simulink model "conSys_2robots_5_vR2014a"  (Simulink 8.3)
settings: Solver=FixedStepDiscrete  StartTime=0.0  StopTime=200  FixedStep=Ts  RelTol=1e-3
values from neighbouring files (symbols this model uses):
  ck = double(max(abs([par.q0_r1;par.q0_r2] - [par.q0r_r1;par.q0r_r2]))*20/7000 + 6)    [startUp_conSys_2robots_1_vGPU_vR2014a.m]    (also in startUp_conSys_2robots_1_vR2014a.m = max(abs([par.q0_r1;par.q0_r2] - [par.q0r_r1;par.q0r_r2]))*20; startUp_conSys_2robots_2_vR2014a.m = max(abs([par.q0_r1;par.q0_r2] - [par.q0r_r1;par.q0r_r2]))*20; startUp_conSys_2robots_3_vR2014a.m = max(abs([par.q0_r1;par.q0_r2] - [par.q0r_r1;par.q0r_r2]))*20; startUp_conSys_2robots_4_vR2014a.m = max(abs([par.q0_r1;par.q0_r2] - [par.q0r_r1;par.q0r_r2]))*20)
  d_0 = 2000    [startUp_conSys_2robots_1_vGPU_vR2014a.m]    (also in startUp_conSys_2robots_1_vR2014a.m = 200; startUp_conSys_2robots_2_vR2014a.m = 200; startUp_conSys_2robots_3_vR2014a.m; startUp_conSys_2robots_4_vR2014a.m = 200)
  do1r_0 = dthc_0 + dph1_0    (= 0.2)    [startUp_conSys_2robots_1_vGPU_vR2014a.m]    (also in startUp_conSys_2robots_1_vR2014a.m = 0; startUp_conSys_2robots_2_vR2014a.m = 0; startUp_conSys_2robots_3_vR2014a.m = 0; startUp_conSys_2robots_4_vR2014a.m = 0)
  do2r_0 = dthc_0 + dph2_0    (= -0.2)    [startUp_conSys_2robots_1_vGPU_vR2014a.m]    (also in startUp_conSys_2robots_1_vR2014a.m = 0; startUp_conSys_2robots_2_vR2014a.m = 0; startUp_conSys_2robots_3_vR2014a.m = 0; startUp_conSys_2robots_4_vR2014a.m = 0)
  dx1r_0 = dxc_0 + sin(thc_0)*dd_0 + d_0*cos(thc_0)*dthc_0    [startUp_conSys_2robots_1_vGPU_vR2014a.m]    (also in startUp_conSys_2robots_1_vR2014a.m; startUp_conSys_2robots_2_vR2014a.m; startUp_conSys_2robots_3_vR2014a.m; startUp_conSys_2robots_4_vR2014a.m)
  dx2r_0 = dxc_0 - sin(thc_0)*dd_0 - d_0*cos(thc_0)*dthc_0    [startUp_conSys_2robots_1_vGPU_vR2014a.m]    (also in startUp_conSys_2robots_1_vR2014a.m; startUp_conSys_2robots_2_vR2014a.m; startUp_conSys_2robots_3_vR2014a.m; startUp_conSys_2robots_4_vR2014a.m)
  dy1r_0 = dyc_0 + cos(thc_0)*dd_0 - d_0*sin(thc_0)*dthc_0    [startUp_conSys_2robots_1_vGPU_vR2014a.m]    (also in startUp_conSys_2robots_1_vR2014a.m; startUp_conSys_2robots_2_vR2014a.m; startUp_conSys_2robots_3_vR2014a.m; startUp_conSys_2robots_4_vR2014a.m)
  dy2r_0 = dyc_0 - cos(thc_0)*dd_0 + d_0*sin(thc_0)*dthc_0    [startUp_conSys_2robots_1_vGPU_vR2014a.m]    (also in startUp_conSys_2robots_1_vR2014a.m; startUp_conSys_2robots_2_vR2014a.m; startUp_conSys_2robots_3_vR2014a.m; startUp_conSys_2robots_4_vR2014a.m)
  o1r_0 = pi/2 - thc_0    (= 0)    [startUp_conSys_2robots_1_vGPU_vR2014a.m]    (also in startUp_conSys_2robots_1_vR2014a.m = pi/2 - thc_0; startUp_conSys_2robots_2_vR2014a.m = pi/2 - thc_0; startUp_conSys_2robots_3_vR2014a.m; startUp_conSys_2robots_4_vR2014a.m = th1_0)
  o2r_0 = pi/2 - thc_0    (= 0)    [startUp_conSys_2robots_1_vGPU_vR2014a.m]    (also in startUp_conSys_2robots_1_vR2014a.m = pi/2 - thc_0; startUp_conSys_2robots_2_vR2014a.m = pi/2 - thc_0; startUp_conSys_2robots_3_vR2014a.m; startUp_conSys_2robots_4_vR2014a.m = th2_0)
  thc_0 = pi/2    (= 1.57079632679)    [startUp_conSys_2robots_1_vGPU_vR2014a.m]    (also in startUp_conSys_2robots_1_vR2014a.m = atan2(1/25,1/12.5) + pi/2; startUp_conSys_2robots_2_vR2014a.m = atan2(1/25,1/12.5) + pi/2; startUp_conSys_2robots_3_vR2014a.m; startUp_conSys_2robots_4_vR2014a.m = atan2(1/25,1/12.5) + pi/2)
  Ts = 1/200    (= 0.005)    [startUp_conSys_2robots_1_vGPU_vR2014a.m]    (also in startUp_conSys_2robots_1_vR2014a.m = 0.0125; startUp_conSys_2robots_2_vR2014a.m = 0.01; startUp_conSys_2robots_3_vR2014a.m; startUp_conSys_2robots_4_vR2014a.m)
  x1_0 = 12000    [startUp_conSys_2robots_1_vGPU_vR2014a.m]    (also in startUp_conSys_2robots_1_vR2014a.m = 13178.9; startUp_conSys_2robots_2_vR2014a.m = 13178.9; startUp_conSys_2robots_3_vR2014a.m; startUp_conSys_2robots_4_vR2014a.m = 13178.9)
  x2_0 = 8000    [startUp_conSys_2robots_1_vGPU_vR2014a.m]    (also in startUp_conSys_2robots_1_vR2014a.m = 12821.1; startUp_conSys_2robots_2_vR2014a.m = 12821.1; startUp_conSys_2robots_3_vR2014a.m; startUp_conSys_2robots_4_vR2014a.m = 12821.1)
  xc_0 = 10000    [startUp_conSys_2robots_1_vGPU_vR2014a.m]    (also in startUp_conSys_2robots_1_vR2014a.m = 13000; startUp_conSys_2robots_2_vR2014a.m = 13000; startUp_conSys_2robots_3_vR2014a.m; startUp_conSys_2robots_4_vR2014a.m = 13000)
  y1_0 = 10000    [startUp_conSys_2robots_1_vGPU_vR2014a.m]    (also in startUp_conSys_2robots_1_vR2014a.m = 12910.6; startUp_conSys_2robots_2_vR2014a.m = 12910.6; startUp_conSys_2robots_3_vR2014a.m; startUp_conSys_2robots_4_vR2014a.m = 12910.6)
  y2_0 = 10000    [startUp_conSys_2robots_1_vGPU_vR2014a.m]    (also in startUp_conSys_2robots_1_vR2014a.m = 13089.4; startUp_conSys_2robots_2_vR2014a.m = 13089.4; startUp_conSys_2robots_3_vR2014a.m; startUp_conSys_2robots_4_vR2014a.m = 13089.4)
  yc_0 = 10000    [startUp_conSys_2robots_1_vGPU_vR2014a.m]    (also in startUp_conSys_2robots_1_vR2014a.m = 13000; startUp_conSys_2robots_2_vR2014a.m = 13000; startUp_conSys_2robots_3_vR2014a.m; startUp_conSys_2robots_4_vR2014a.m = 13000)
undefined symbols (not defined in the file or in its folder): absoluteAngle01_vR2014a, absoluteAngle02_vR2014a, absoluteAngle03_vR2014a, absoluteAngle04_vR2014a, absoluteAngle05_vR2014a, absoluteAngle06_vR2014a, absoluteAngle07_vR2014a, DiscIntNeverNeededParam
undefined symbols (not defined in the file): ADAMS_cwd, ADAMS_exec, ADAMS_host, ADAMS_init, ADAMS_inputs, ADAMS_outputs, ADAMS_prefix, ADAMS_static, ADAMS_sysdir
libraries: simulink x18, cstblocks x1
(part 1 of 2)
settings Model: Creator=baqumau  LastModifiedBy=mauro
settings DataIOCC: SignalLoggingSaveFormat=Dataset
settings DebuggingCC: UnderspecifiedInitializationDetection=Simplified  StateNameClashWarn=none
settings GRTTargetCC: CombineOutputUpdateFcns=on  GRTInterface=off

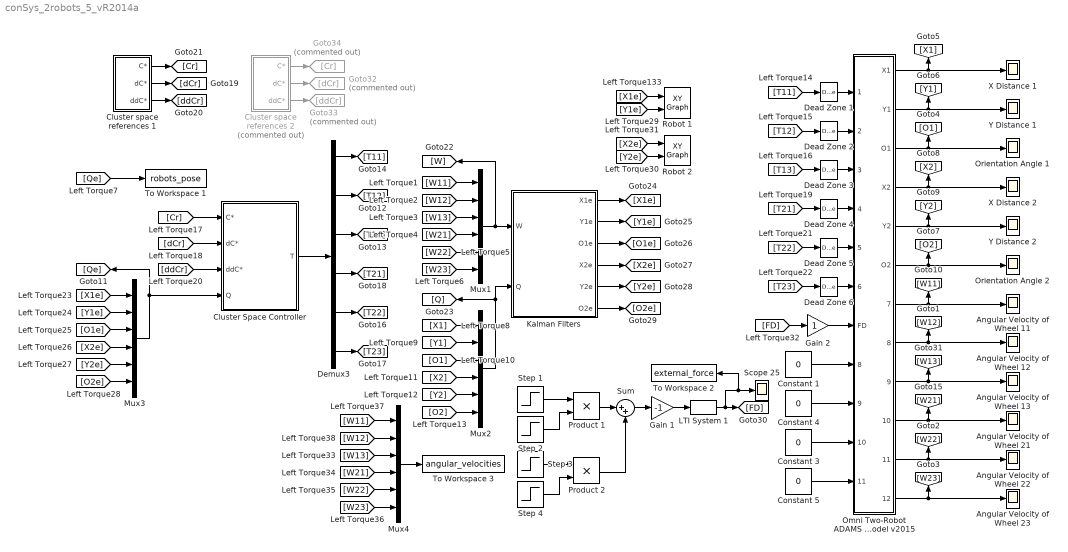
== system conSys_2robots_5_vR2014a ==
  Angular Velocity of Wheel {11..13,21..23} (6 alike) : Scope
      Angular Velocity of Wheel 11 settings: YMin=-20  YMax=20  SaveName=ScopeData3
      Angular Velocity of Wheel 12 settings: YMin=-200  YMax=20  SaveName=ScopeData6
      Angular Velocity of Wheel 13 settings: YMin=-10  YMax=20  SaveName=ScopeData9
      Angular Velocity of Wheel 21 settings: YMin=-20  YMax=20  SaveName=ScopeData2
      Angular Velocity of Wheel 22 settings: YMin=-15  YMax=18  SaveName=ScopeData10
      Angular Velocity of Wheel 23 settings: YMin=-15  YMax=15  SaveName=ScopeData11
  Cluster Space Controller : Subsystem
  Cluster space references 1 : Subsystem
  Cluster space references 2 : Subsystem  Commented=on
  Constant {1,3..5} (4 alike) : Constant  Value=0
  Dead Zone {1..6} (6 alike) : DeadZone  LowerValue=-25  UpperValue=25  SaturateOnIntegerOverflow=on
  Demux3 : Demux  Outputs=6
  Gain 1 : Gain  Gain=-1
  Gain 2 : Gain
  Goto32 : Goto  Commented=on  GotoTag=dCr
  Goto33 : Goto  Commented=on  GotoTag=ddCr
  Goto34 : Goto  Commented=on  GotoTag=Cr
  Kalman Filters : Subsystem
  LTI System 1 : cstblocks/LTI System  sys=Fz  IC=[]
  Mux{1..4} (4 alike) : Mux  Inputs=6
  Omni Two-Robot ADAMS Model v2015 : Subsystem
  Orientation Angle 1 : Scope
  Orientation Angle 2 : Scope
      settings: YMin=-3  YMax=3  SaveName=ScopeData12
  Product 1 : Product
  Product 2 : Product
  Robot 1 : simulink/Sinks/XY Graph  xmin=0  xmax=20000  ymin=0  ymax=20000  st=-1
  Robot 2 : simulink/Sinks/XY Graph  xmin=0  xmax=20000  ymin=0  ymax=20000  st=-1
  Scope 25 : Scope
      settings: YMin=-6  YMax=6  SaveName=ScopeData36
  Step 1 : Step  Time=60  SampleTime=0
  Step 2 : Step  Time=100  Before=1  After=0  SampleTime=0
  Step 3 : Step  Time=130  After=-1  SampleTime=0
  Step 4 : Step  Time=170  Before=1  After=0  SampleTime=0
  Sum : Sum  Inputs=|++
  To Workspace 1 : ToWorkspace  VariableName=robots_pose  SaveFormat=Structure With Time  SampleTime=-1
  To Workspace 2 : ToWorkspace  VariableName=external_force  SaveFormat=Structure With Time  SampleTime=-1
  To Workspace 3 : ToWorkspace  VariableName=angular_velocities  SaveFormat=Structure With Time  SampleTime=-1
  X Distance 1 : Scope
      settings: YMin=0  YMax=20000  SaveName=ScopeData4
  X Distance 2 : Scope
      settings: YMin=0  YMax=20000  SaveName=ScopeData16
  Y Distance 1 : Scope
      settings: YMin=0  YMax=20000
  Y Distance 2 : Scope
      settings: YMin=0  YMax=20000  SaveName=ScopeData17
  wires:
  Omni Two-Robot ADAMS Model v2015/1(X1) -> X Distance 1/1, [X1]
  Omni Two-Robot ADAMS Model v2015/2(Y1) -> [Y1], Y Distance 1/1
  Omni Two-Robot ADAMS Model v2015/3(O1) -> [O1], Orientation Angle 1/1
  Omni Two-Robot ADAMS Model v2015/7(W11) -> [W11], Angular Velocity of Wheel 11/1
  Omni Two-Robot ADAMS Model v2015/10(W21) -> [W21], Angular Velocity of Wheel 21/1
  Omni Two-Robot ADAMS Model v2015/9(W13) -> Angular Velocity of Wheel 13/1, [W13]
  Omni Two-Robot ADAMS Model v2015/4(X2) -> X Distance 2/1, [X2]
  Omni Two-Robot ADAMS Model v2015/5(Y2) -> Y Distance 2/1, [Y2]
  Omni Two-Robot ADAMS Model v2015/6(O2) -> Orientation Angle 2/1, [O2]
  Omni Two-Robot ADAMS Model v2015/8(W12) -> Angular Velocity of Wheel 12/1, [W12]
  Omni Two-Robot ADAMS Model v2015/11(W22) -> Angular Velocity of Wheel 22/1, [W22]
  Omni Two-Robot ADAMS Model v2015/12(W23) -> [W23], Angular Velocity of Wheel 23/1
  [O1e] -> Mux3/3
  [X2e] -> Mux3/4
  [Y2e] -> Mux3/5
  [O2e] -> Mux3/6
  [X1e] -> Mux3/1
  [Y1e] -> Mux3/2
  [Cr] -> Cluster Space Controller/1(C*)
  [dCr] -> Cluster Space Controller/2(dC*)
  Mux3/1 -> Cluster Space Controller/4(Q), [Qe]
  Cluster Space Controller/1(T) -> Demux3/1
  Demux3/1 -> [T11]
  Demux3/2 -> [T12]
  Demux3/3 -> [T13]
  Demux3/4 -> [T21]
  Demux3/5 -> [T22]
  Demux3/6 -> [T23]
  Cluster space references 1/1(C*) -> [Cr]
  Cluster space references 1/2(dC*) -> [dCr]
  Cluster space references 1/3(ddC*) -> [ddCr]
  [ddCr] -> Cluster Space Controller/3(ddC*)
  [W13] -> Mux1/3
  [W21] -> Mux1/4
  [W22] -> Mux1/5
  [W23] -> Mux1/6
  [W11] -> Mux1/1
  [W12] -> Mux1/2
  Mux1/1 -> Kalman Filters/1(W), [W]
  [Qe] -> To Workspace 1/1
  [O1] -> Mux2/3
  [X2] -> Mux2/4
  [Y2] -> Mux2/5
  [O2] -> Mux2/6
  [X1] -> Mux2/1
  [Y1] -> Mux2/2
  Kalman Filters/1(X1e) -> [X1e]
  Kalman Filters/2(Y1e) -> [Y1e]
  Kalman Filters/3(O1e) -> [O1e]
  Kalman Filters/4(X2e) -> [X2e]
  Kalman Filters/5(Y2e) -> [Y2e]
  Kalman Filters/6(O2e) -> [O2e]
  [T11] -> Dead Zone 1/1
  [T12] -> Dead Zone 2/1
  [T13] -> Dead Zone 3/1
  [T21] -> Dead Zone 4/1
  [T22] -> Dead Zone 5/1
  [T23] -> Dead Zone 6/1
  [FD] -> Gain 2/1
  Constant 1/1 -> Omni Two-Robot ADAMS Model v2015/8(FX1)
  Constant 3/1 -> Omni Two-Robot ADAMS Model v2015/10(FY1)
  Constant 4/1 -> Omni Two-Robot ADAMS Model v2015/9(FX2)
  Constant 5/1 -> Omni Two-Robot ADAMS Model v2015/11(FY2)
  [X1e] -> Robot 1/1
  [Y1e] -> Robot 1/2
  [X2e] -> Robot 2/1
  [Y2e] -> Robot 2/2
  Step 1/1 -> Product 1/1
  Step 2/1 -> Product 1/2
  Step 3/1 -> Product 2/1
  Step 4/1 -> Product 2/2
  Product 1/1 -> Sum/1
  Product 2/1 -> Sum/2
  Sum/1 -> Gain 1/1
  LTI System 1/1 -> To Workspace 2/1, Scope 25/1, [FD]
  Gain 1/1 -> LTI System 1/1
  Cluster space references 2/1(C*) -> Goto34/1
  Cluster space references 2/2(dC*) -> Goto32/1
  Cluster space references 2/3(ddC*) -> Goto33/1
  [W13] -> Mux4/3
  [W21] -> Mux4/4
  [W22] -> Mux4/5
  [W23] -> Mux4/6
  [W11] -> Mux4/1
  [W12] -> Mux4/2
  Mux4/1 -> To Workspace 3/1
  Mux2/1 -> Kalman Filters/2(Q), [Q]
  Gain 2/1 -> Omni Two-Robot ADAMS Model v2015/7(FD)
  Dead Zone 1/1 -> Omni Two-Robot ADAMS Model v2015/1(T11)
  Dead Zone 2/1 -> Omni Two-Robot ADAMS Model v2015/2(T12)
  Dead Zone 3/1 -> Omni Two-Robot ADAMS Model v2015/3(T13)
  Dead Zone 4/1 -> Omni Two-Robot ADAMS Model v2015/4(T21)
  Dead Zone 5/1 -> Omni Two-Robot ADAMS Model v2015/5(T22)
  Dead Zone 6/1 -> Omni Two-Robot ADAMS Model v2015/6(T23)

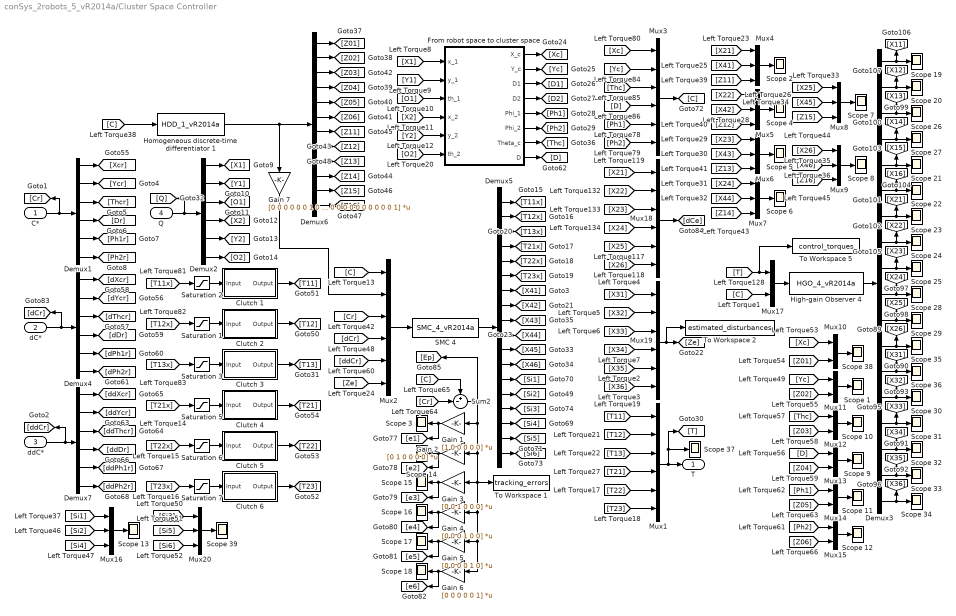
== system conSys_2robots_5_vR2014a/Cluster Space Controller ==
  C* : Inport
  dC* : Inport  Port=2
  ddC* : Inport  Port=3
  Q : Inport  Port=4
  Clutch 1 : Subsystem
  Clutch 2 : Subsystem
  Clutch 3 : Subsystem
  Clutch 4 : Subsystem
  Clutch 5 : Subsystem
  Clutch 6 : Subsystem
  Demux{1..2,4,7} (4 alike) : Demux  Outputs=6
  Demux3 : Demux  Outputs=18
  Demux5 : Demux  Outputs=18
  Demux6 : Demux  Outputs=12
  From robot space to cluster space : Subsystem
  Gain 1 : Gain  Gain=[1 0 0 0 0 0]  Multiplication=Matrix(K*u)
  Gain 2 : Gain  Gain=[0 1 0 0 0 0]  Multiplication=Matrix(K*u)
  Gain 3 : Gain  Gain=[0 0 1 0 0 0]  Multiplication=Matrix(K*u)
  Gain 4 : Gain  Gain=[0 0 0 1 0 0]  Multiplication=Matrix(K*u)
  Gain 5 : Gain  Gain=[0 0 0 0 1 0]  Multiplication=Matrix(K*u)
  Gain 6 : Gain  Gain=[0 0 0 0 0 1]  Multiplication=Matrix(K*u)
  Gain 7 : Gain  Gain=[0 0 0 0 0 0 1 0 0 0 0 0;0 0 0 0 0 0 0 1 0 0 0 0;0 0 0 0 0 0 0 0 1 0 0 0;0 0 0 0 0 0 0 0 0 1 0 0;0 0 0 0 0 0 0 0 0 0 1 0;0 0 0 0 0 0 0 0 0 0 0 1]  Multiplication=Matrix(K*u)
  High-gain Observer 4 : S-Function  FunctionName=HGO_4_vR2014a  Parameters=par  EnableBusSupport=off
  Homogeneous discrete-time differentiator 1 : S-Function  FunctionName=HDD_1_vR2014a  Parameters=par  EnableBusSupport=off
  Mux{1..3,18..19} (5 alike) : Mux  Inputs=6
  Mux{10..15,17} (7 alike) : Mux  Inputs=2
  Mux{4..9,16,20} (8 alike) : Mux  Inputs=3
  SMC 4 : S-Function  FunctionName=SMC_4_vR2014a  Parameters=par  EnableBusSupport=off
  Saturation {1..3,5..7} (6 alike) : Saturate  UpperLimit=100  LowerLimit=-100
  Scope {1..39} (39 alike) : Scope
      Scope 1 settings: YMin=0  YMax=15000  SaveName=ScopeData21
      Scope 10 settings: SaveName=ScopeData39
      Scope 11 settings: SaveName=ScopeData43
      Scope 12 settings: SaveName=ScopeData44
      Scope 13 settings: YMin=-2000  YMax=1000  SaveName=ScopeData45
      Scope 14 settings: YMin=-5000  YMax=1000  SaveName=ScopeData77
      Scope 15 settings: YMin=-4  YMax=4  SaveName=ScopeData78
      Scope 16 settings: YMin=-2000  YMax=2000  SaveName=ScopeData82
      Scope 17 settings: SaveName=ScopeData83
      Scope 18 settings: SaveName=ScopeData84
      Scope 19 settings: YMin=-2000  YMax=16000  SaveName=ScopeData86
      Scope 2 settings: YMin=0  YMax=140  SaveName=ScopeData22
      Scope 20 settings: YMin=0  YMax=20000  SaveName=ScopeData87
      Scope 21 settings: YMin=0  YMax=5000  SaveName=ScopeData88
      Scope 22 settings: YMin=-100  YMax=200  SaveName=ScopeData90
      Scope 23 settings: YMin=-10  YMax=100  SaveName=ScopeData91
      Scope 24 settings: YMin=-50  YMax=50  SaveName=ScopeData92
      Scope 25 settings: YMin=-6  YMax=6  SaveName=ScopeData93
      Scope 26 settings: SaveName=ScopeData94
      Scope 27 settings: TimeRange=388  YMin=-1000  YMax=1000  SaveName=ScopeData95
      Scope 28 settings: YMin=-5000  YMax=1000  SaveName=ScopeData96
      Scope 29 settings: YMin=-10  YMax=10  SaveName=ScopeData97
      Scope 3 settings: YMin=-5000  YMax=3000  SaveName=ScopeData40
      Scope 30 settings: YMin=-1000  YMax=1000  SaveName=ScopeData98
      Scope 31 settings: YMin=-2  YMax=2  SaveName=ScopeData99
      Scope 32 settings: YMin=-1000  YMax=500  SaveName=ScopeData100
      Scope 33 settings: YMin=-6  YMax=8  SaveName=ScopeData101
      Scope 34 settings: YMin=-4  YMax=4  SaveName=ScopeData102
      Scope 35 settings: SaveName=ScopeData103
      Scope 36 settings: YMin=-1000  YMax=500  SaveName=ScopeData104
      Scope 37 settings: YMin=-100  YMax=100  SaveName=ScopeData119
      Scope 38 settings: YMin=0  YMax=15000  SaveName=ScopeData46
      Scope 39 settings: YMin=-15  YMax=15  SaveName=ScopeData47
      Scope 4 settings: YMin=-100  YMax=100  SaveName=ScopeData23
      Scope 5 settings: YMin=-1  YMax=1  SaveName=ScopeData24
      Scope 6 settings: YMin=-1000  YMax=1000  SaveName=ScopeData30
      Scope 7 settings: SaveName=ScopeData31
      Scope 8 settings: YMin=-10  YMax=10  SaveName=ScopeData37
      Scope 9 settings: YMin=500  YMax=10000  SaveName=ScopeData41
  Sum2 : Sum  Inputs=+-|
  To Workspace 1 : ToWorkspace  VariableName=tracking_errors  SaveFormat=Structure With Time  SampleTime=-1
  To Workspace 2 : ToWorkspace  VariableName=estimated_disturbances  SaveFormat=Structure With Time  SampleTime=-1
  To Workspace 5 : ToWorkspace  VariableName=control_torques  SaveFormat=Structure With Time  SampleTime=-1
  T : Outport
  wires:
  Q/1 -> Demux2/1, [Q]
  Demux2/1 -> [X1]
  Demux2/2 -> [Y1]
  Demux2/3 -> [O1]
  Demux2/4 -> [X2]
  Demux2/5 -> [Y2]
  Demux2/6 -> [O2]
  Mux2/1 -> SMC 4/1
  Demux5/1 -> [T11x]
  Demux5/2 -> [T12x]
  Demux5/3 -> [T13x]
  SMC 4/1 -> Demux5/1
  Demux5/4 -> [T21x]
  Demux5/5 -> [T22x]
  Demux5/6 -> [T23x]
  [Cr] -> Sum2/2
  [C] -> Sum2/1
  [T11x] -> Saturation 2/1
  Clutch 1/1(Output) -> [T11]
  [T12x] -> Saturation 1/1
  Clutch 2/1(Output) -> [T12]
  [T13x] -> Saturation 3/1
  Clutch 3/1(Output) -> [T13]
  [T21x] -> Saturation 5/1
  Clutch 4/1(Output) -> [T21]
  [T22x] -> Saturation 6/1
  Clutch 5/1(Output) -> [T22]
  [T23x] -> Saturation 7/1
  Clutch 6/1(Output) -> [T23]
  [T11] -> Mux1/1
  [T23] -> Mux1/6
  [T21] -> Mux1/4
  [T22] -> Mux1/5
  [T12] -> Mux1/2
  [T13] -> Mux1/3
  Mux1/1 -> [T], Scope 37/1, T/1
  C*/1 -> [Cr], Demux1/1
  Demux1/1 -> [Xcr]
  Demux1/2 -> [Ycr]
  Demux1/3 -> [Thcr]
  Demux1/4 -> [Dr]
  Demux1/5 -> [Ph1r]
  Demux1/6 -> [Ph2r]
  dC*/1 -> [dCr], Demux4/1
  Demux4/1 -> [dXcr]
  Demux4/2 -> [dYcr]
  Demux4/3 -> [dThcr]
  Demux4/4 -> [dDr]
  Demux4/5 -> [dPh1r]
  Demux4/6 -> [dPh2r]
  Demux7/1 -> [ddXcr]
  Demux7/2 -> [ddYcr]
  Demux7/3 -> [ddThcr]
  Demux7/4 -> [ddDr]
  Demux7/5 -> [ddPh1r]
  Demux7/6 -> [ddPh2r]
  ddC*/1 -> [ddCr], Demux7/1
  [Xc] -> Mux3/1
  [Ph2] -> Mux3/6
  [D] -> Mux3/4
  [Ph1] -> Mux3/5
  [Yc] -> Mux3/2
  [Thc] -> Mux3/3
  Mux3/1 -> [C]
  Gain 1/1 -> [e1], Scope 3/1
  Gain 2/1 -> [e2], Scope 14/1
  Gain 3/1 -> [e3], Scope 15/1
  Gain 4/1 -> [e4], Scope 16/1
  Gain 5/1 -> [e5], Scope 17/1
  Sum2/1 -> [Ep], To Workspace 1/1, Gain 6/1, Gain 5/1, Gain 4/1, Gain 3/1, Gain 2/1, Gain 1/1
  Gain 6/1 -> [e6], Scope 18/1
  Mux17/1 -> High-gain Observer 4/1
  Demux3/9 -> Scope 25/1, [X23]
  Demux3/7 -> [X21], Scope 23/1
  Demux3/8 -> [X22], Scope 24/1
  Demux3/5 -> [X15], Scope 21/1
  Demux3/6 -> [X16], Scope 22/1
  High-gain Observer 4/1 -> Demux3/1
  Demux3/3 -> Scope 26/1, [X13]
  Demux3/4 -> Scope 27/1, [X14]
  Demux3/1 -> Scope 19/1, [X11]
  Demux3/2 -> Scope 20/1, [X12]
  Demux3/17 -> Scope 33/1, [X35]
  Demux3/13 -> [X31], Scope 36/1
  Demux3/12 -> [X26], Scope 35/1
  Demux3/18 -> [X36], Scope 34/1
  Demux3/15 -> Scope 31/1, [X33]
  Demux3/10 -> [X24], Scope 28/1
  Demux3/11 -> [X25], Scope 29/1
  Demux3/16 -> Scope 32/1, [X34]
  Demux3/14 -> Scope 30/1, [X32]
  [X21] -> Mux18/1
  [X26] -> Mux18/6
  [X24] -> Mux18/4
  [X25] -> Mux18/5
  [X22] -> Mux18/2
  [X23] -> Mux18/3
  Mux18/1 -> [dCe]
  [T] -> To Workspace 5/1, Mux17/1
  [C] -> Mux17/2
  [X31] -> Mux19/1
  [X36] -> Mux19/6
  [X34] -> Mux19/4
  [X35] -> Mux19/5
  [X32] -> Mux19/2
  [X33] -> Mux19/3
  Mux19/1 -> To Workspace 2/1, [Ze]
  From robot space to cluster space/8(D) -> [D]
  From robot space to cluster space/7(Theta_c) -> [Thc]
  From robot space to cluster space/6(Phi_2) -> [Ph2]
  From robot space to cluster space/5(Phi_1) -> [Ph1]
  From robot space to cluster space/4(D2) -> [D2]
  From robot space to cluster space/3(D1) -> [D1]
  From robot space to cluster space/2(Y_c) -> [Yc]
  From robot space to cluster space/1(X_c) -> [Xc]
  [X1] -> From robot space to cluster space/1(x_1)
  [Y1] -> From robot space to cluster space/2(y_1)
  [O1] -> From robot space to cluster space/3(th_1)
  [X2] -> From robot space to cluster space/4(x_2)
  [Y2] -> From robot space to cluster space/5(y_2)
  [O2] -> From robot space to cluster space/6(th_2)
  [C] -> Mux2/1
  Demux5/7 -> [X41]
  Demux5/8 -> [X42]
  Demux5/9 -> [X43]
  Demux5/10 -> [X44]
  Demux5/11 -> [X45]
  Demux5/12 -> [X46]
  [X21] -> Mux4/1
  [X41] -> Mux4/2
  [X22] -> Mux5/1
  [X42] -> Mux5/2
  [X23] -> Mux6/1
  [X43] -> Mux6/2
  [X24] -> Mux7/1
  [X44] -> Mux7/2
  Mux4/1 -> Scope 2/1
  Mux5/1 -> Scope 4/1
  Mux6/1 -> Scope 5/1
  Mux7/1 -> Scope 6/1
  [X25] -> Mux8/1
  [X45] -> Mux8/2
  Mux8/1 -> Scope 7/1
  [X26] -> Mux9/1
  [X46] -> Mux9/2
  Mux9/1 -> Scope 8/1
  Homogeneous discrete-time differentiator 1/1 -> Demux6/1, Gain 7/1
  [Cr] -> Mux2/3
  [dCr] -> Mux2/4
  [ddCr] -> Mux2/5
  [Ze] -> Mux2/6
  [C] -> Homogeneous discrete-time differentiator 1/1
  Demux6/1 -> [Z01]
  Demux6/2 -> [Z02]
  Demux6/3 -> [Z03]
  Demux6/4 -> [Z04]
  Demux6/5 -> [Z05]
  Demux6/6 -> [Z06]
  Demux6/7 -> [Z11]
  Demux6/8 -> [Z12]
  Demux6/9 -> [Z13]
  Demux6/10 -> [Z14]
  Demux6/11 -> [Z15]
  Demux6/12 -> [Z16]
  [Z11] -> Mux4/3
  [Z12] -> Mux5/3
  [Z13] -> Mux6/3
  [Z14] -> Mux7/3
  [Z15] -> Mux8/3
  [Z16] -> Mux9/3
  [Xc] -> Mux10/1
  Mux10/1 -> Scope 38/1
  [Z01] -> Mux10/2
  [Yc] -> Mux11/1
  Mux11/1 -> Scope 1/1
  [Z02] -> Mux11/2
  [Thc] -> Mux12/1
  Mux12/1 -> Scope 10/1
  [Z03] -> Mux12/2
  [D] -> Mux13/1
  Mux13/1 -> Scope 9/1
  [Z04] -> Mux13/2
  [Ph1] -> Mux14/1
  Mux14/1 -> Scope 11/1
  [Z05] -> Mux14/2
  [Ph2] -> Mux15/1
  Mux15/1 -> Scope 12/1
  [Z06] -> Mux15/2
  Gain 7/1 -> Mux2/2
  Saturation 1/1 -> Clutch 2/1(Input)
  Saturation 2/1 -> Clutch 1/1(Input)
  Saturation 3/1 -> Clutch 3/1(Input)
  Saturation 5/1 -> Clutch 4/1(Input)
  Saturation 6/1 -> Clutch 5/1(Input)
  Saturation 7/1 -> Clutch 6/1(Input)
  Demux5/13 -> [Si1]
  Demux5/14 -> [Si2]
  Demux5/15 -> [Si3]
  Demux5/16 -> [Si4]
  Demux5/17 -> [Si5]
  Demux5/18 -> [Si6]
  [Si1] -> Mux16/1
  Mux16/1 -> Scope 13/1
  [Si2] -> Mux16/2
  [Si4] -> Mux16/3
  [Si3] -> Mux20/1
  Mux20/1 -> Scope 39/1
  [Si5] -> Mux20/2
  [Si6] -> Mux20/3

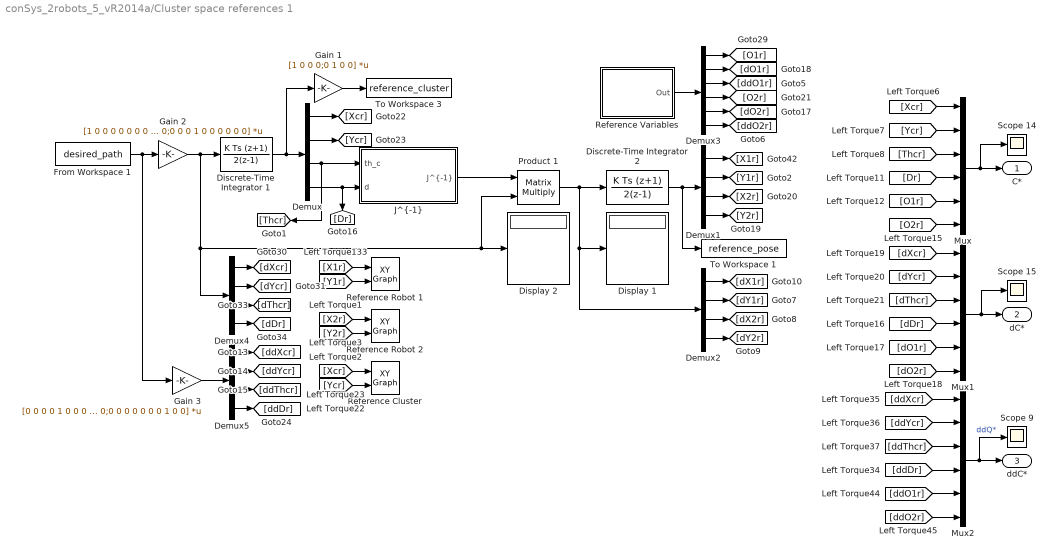
== system conSys_2robots_5_vR2014a/Cluster space references 1 ==
  Demux{,1..2,4..5} (5 alike) : Demux
  Demux3 : Demux  Outputs=6
  Discrete-Time Integrator 1 : DiscreteIntegrator  IntegratorMethod=Integration: Trapezoidal  InitialCondition=[xc_0 yc_0 thc_0 d_0]'  SampleTime=Ts  ICPrevOutput=DiscIntNeverNeededParam  ICPrevScaledInput=DiscIntNeverNeededParam
  Discrete-Time Integrator 2 : DiscreteIntegrator  IntegratorMethod=Integration: Trapezoidal  InitialCondition=[x1_0 y1_0 x2_0 y2_0]'  SampleTime=Ts  ICPrevOutput=DiscIntNeverNeededParam  ICPrevScaledInput=DiscIntNeverNeededParam
  Display 1 : Display
  Display 2 : Display
  From Workspace 1 : FromWorkspace  VariableName=desired_path  SampleTime=Ts  OutputAfterFinalValue=Holding final value
  Gain 1 : Gain  Gain=[1 0 0 0;0 1 0 0]  Multiplication=Matrix(K*u)
  Gain 2 : Gain  Gain=[1 0 0 0 0 0 0 0 0 0;0 1 0 0 0 0 0 0 0 0;0 0 1 0 0 0 0 0 0 0;0 0 0 1 0 0 0 0 0 0]  Multiplication=Matrix(K*u)
  Gain 3 : Gain  Gain=[0 0 0 0 1 0 0 0 0 0;0 0 0 0 0 1 0 0 0 0;0 0 0 0 0 0 1 0 0 0;0 0 0 0 0 0 0 1 0 0]  Multiplication=Matrix(K*u)
  "J^{-1}" : Subsystem
  Mux : Mux  Inputs=6
  Mux1 : Mux  Inputs=6
  Mux2 : Mux  Inputs=6
  Product 1 : Product  Multiplication=Matrix(*)
  Reference Cluster : simulink/Sinks/XY Graph  xmin=0  xmax=20000  ymin=0  ymax=20000  st=-1
  Reference Robot 1 : simulink/Sinks/XY Graph  xmin=0  xmax=20000  ymin=0  ymax=20000  st=-1
  Reference Robot 2 : simulink/Sinks/XY Graph  xmin=0  xmax=20000  ymin=0  ymax=20000  st=-1
  Reference Variables : Subsystem
  Scope 14 : Scope
      settings: ShowLegends=on  TimeRange=200  YMin=-1000  YMax=14000  SaveName=ScopeData59
  Scope 15 : Scope
      settings: ShowLegends=on  TimeRange=500  YMin=-1  YMax=1  SaveName=ScopeData69
  Scope 9 : Scope
      settings: ShowLegends=on  TimeRange=500  YMin=-0.15  YMax=0.15  SaveName=ScopeData80
  To Workspace 1 : ToWorkspace  VariableName=reference_pose  SaveFormat=Structure With Time  SampleTime=-1
  To Workspace 3 : ToWorkspace  VariableName=reference_cluster  SaveFormat=Structure With Time  SampleTime=-1
  C* : Outport
  dC* : Outport  Port=2
  ddC* : Outport  Port=3
  wires:
  Demux4/1 -> [dXcr]
  Demux4/2 -> [dYcr]
  Demux4/4 -> [dDr]
  Demux4/3 -> [dThcr]
  "J^{-1}"/1("J^{-1}") -> Product 1/1
  Product 1/1 -> Demux2/1, Display 1/1, Discrete-Time Integrator 2/1
  [X1r] -> Reference Robot 1/1
  [Y1r] -> Reference Robot 1/2
  [X2r] -> Reference Robot 2/1
  [Y2r] -> Reference Robot 2/2
  From Workspace 1/1 -> Gain 3/1, Gain 2/1
  Discrete-Time Integrator 2/1 -> To Workspace 1/1, Demux1/1
  Demux1/1 -> [X1r]
  Demux1/2 -> [Y1r]
  Demux1/3 -> [X2r]
  Demux1/4 -> [Y2r]
  Reference Variables/1(Out) -> Demux3/1
  Demux3/1 -> [O1r]
  Demux3/2 -> [dO1r]
  Discrete-Time Integrator 1/1 -> Gain 1/1, Demux/1
  Demux/1 -> [Xcr]
  Demux/2 -> [Ycr]
  Demux/3 -> [Thcr], "J^{-1}"/1(th_c)
  Demux/4 -> [Dr], "J^{-1}"/2(d)
  Gain 1/1 -> To Workspace 3/1
  [Dr] -> Mux/4
  [Thcr] -> Mux/3
  [Ycr] -> Mux/2
  [O1r] -> Mux/5
  [Xcr] -> Mux/1
  [O2r] -> Mux/6
  [dDr] -> Mux1/4
  [dXcr] -> Mux1/1
  [dThcr] -> Mux1/3
  [dO2r] -> Mux1/6
  [dO1r] -> Mux1/5
  [dYcr] -> Mux1/2
  Mux/1 -> Scope 14/1, C*/1
  Mux1/1 -> Scope 15/1, dC*/1
  [Xcr] -> Reference Cluster/1
  [Ycr] -> Reference Cluster/2
  Demux2/1 -> [dX1r]
  Demux2/2 -> [dY1r]
  Demux2/3 -> [dX2r]
  Demux2/4 -> [dY2r]
  Mux2/1 -> ddC*/1, Scope 9/1  "ddQ*"
  [ddXcr] -> Mux2/1
  [ddYcr] -> Mux2/2
  [ddThcr] -> Mux2/3
  [ddDr] -> Mux2/4
  [ddO1r] -> Mux2/5
  [ddO2r] -> Mux2/6
  Gain 2/1 -> Demux4/1, Product 1/2, Display 2/1, Discrete-Time Integrator 1/1
  Gain 3/1 -> Demux5/1
  Demux5/1 -> [ddXcr]
  Demux5/2 -> [ddYcr]
  Demux5/3 -> [ddThcr]
  Demux5/4 -> [ddDr]
  Demux3/4 -> [O2r]
  Demux3/5 -> [dO2r]
  Demux3/3 -> [ddO1r]
  Demux3/6 -> [ddO2r]

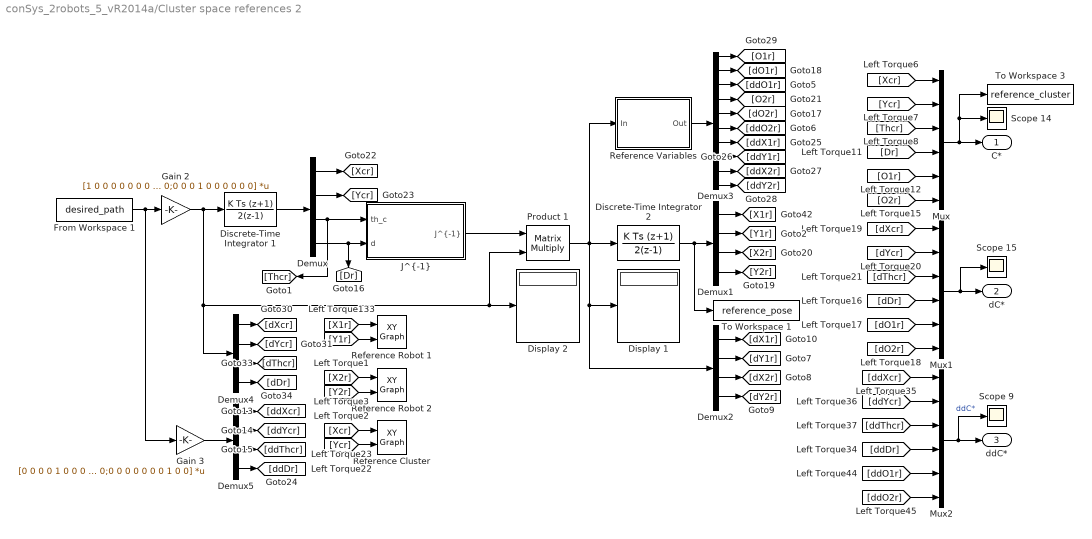
== system conSys_2robots_5_vR2014a/Cluster space references 2 ==
  Demux{,1..2,4..5} (5 alike) : Demux
  Demux3 : Demux  Outputs=10
  Discrete-Time Integrator 1 : DiscreteIntegrator  IntegratorMethod=Integration: Trapezoidal  InitialCondition=[xc_0 yc_0 thc_0 d_0]'  SampleTime=Ts  ICPrevOutput=DiscIntNeverNeededParam  ICPrevScaledInput=DiscIntNeverNeededParam
  Discrete-Time Integrator 2 : DiscreteIntegrator  IntegratorMethod=Integration: Trapezoidal  InitialCondition=[x1_0 y1_0 x2_0 y2_0]'  SampleTime=Ts  ICPrevOutput=DiscIntNeverNeededParam  ICPrevScaledInput=DiscIntNeverNeededParam
  Display 1 : Display
  Display 2 : Display
  From Workspace 1 : FromWorkspace  VariableName=desired_path  SampleTime=Ts  OutputAfterFinalValue=Holding final value
  Gain 2 : Gain  Gain=[1 0 0 0 0 0 0 0 0 0;0 1 0 0 0 0 0 0 0 0;0 0 1 0 0 0 0 0 0 0;0 0 0 1 0 0 0 0 0 0]  Multiplication=Matrix(K*u)
  Gain 3 : Gain  Gain=[0 0 0 0 1 0 0 0 0 0;0 0 0 0 0 1 0 0 0 0;0 0 0 0 0 0 1 0 0 0;0 0 0 0 0 0 0 1 0 0]  Multiplication=Matrix(K*u)
  "J^{-1}" : Subsystem
  Mux : Mux  Inputs=6
  Mux1 : Mux  Inputs=6
  Mux2 : Mux  Inputs=6
  Product 1 : Product  Multiplication=Matrix(*)
  Reference Cluster : simulink/Sinks/XY Graph  xmin=0  xmax=20000  ymin=0  ymax=20000  st=-1
  Reference Robot 1 : simulink/Sinks/XY Graph  xmin=0  xmax=20000  ymin=0  ymax=20000  st=-1
  Reference Robot 2 : simulink/Sinks/XY Graph  xmin=0  xmax=20000  ymin=0  ymax=20000  st=-1
  Reference Variables : Subsystem
  Scope 14 : Scope
      settings: ShowLegends=on  TimeRange=500  YMin=-6  YMax=0  SaveName=ScopeData59
  Scope 15 : Scope
      settings: ShowLegends=on  TimeRange=500  YMin=-1  YMax=1  SaveName=ScopeData69
  Scope 9 : Scope
      settings: ShowLegends=on  TimeRange=500  YMin=-0.15  YMax=0.15  SaveName=ScopeData80
  To Workspace 1 : ToWorkspace  VariableName=reference_pose  SaveFormat=Structure With Time  SampleTime=-1
  To Workspace 3 : ToWorkspace  VariableName=reference_cluster  SaveFormat=Structure With Time  SampleTime=-1
  C* : Outport
  dC* : Outport  Port=2
  ddC* : Outport  Port=3
  wires:
  Demux3/10 -> [ddY2r]
  Demux3/9 -> [ddX2r]
  Demux3/8 -> [ddY1r]
  Demux3/7 -> [ddX1r]
  Demux3/6 -> [ddO2r]
  Demux3/3 -> [ddO1r]
  Demux3/5 -> [dO2r]
  Demux3/4 -> [O2r]
  Demux5/4 -> [ddDr]
  Demux5/3 -> [ddThcr]
  Demux5/2 -> [ddYcr]
  Demux5/1 -> [ddXcr]
  Gain 3/1 -> Demux5/1
  Gain 2/1 -> Discrete-Time Integrator 1/1, Display 2/1, Product 1/2, Demux4/1
  [ddO2r] -> Mux2/6
  [ddO1r] -> Mux2/5
  [ddDr] -> Mux2/4
  [ddThcr] -> Mux2/3
  [ddYcr] -> Mux2/2
  [ddXcr] -> Mux2/1
  Mux2/1 -> Scope 9/1, ddC*/1  "ddC*"
  Demux2/4 -> [dY2r]
  Demux2/3 -> [dX2r]
  Demux2/2 -> [dY1r]
  Demux2/1 -> [dX1r]
  [Ycr] -> Reference Cluster/2
  [Xcr] -> Reference Cluster/1
  Mux1/1 -> dC*/1, Scope 15/1
  Mux/1 -> C*/1, To Workspace 3/1, Scope 14/1
  [dYcr] -> Mux1/2
  [dO1r] -> Mux1/5
  [dO2r] -> Mux1/6
  [dThcr] -> Mux1/3
  [dXcr] -> Mux1/1
  [dDr] -> Mux1/4
  [O2r] -> Mux/6
  [Xcr] -> Mux/1
  [O1r] -> Mux/5
  [Ycr] -> Mux/2
  [Thcr] -> Mux/3
  [Dr] -> Mux/4
  Discrete-Time Integrator 1/1 -> Demux/1
  Demux/4 -> "J^{-1}"/2(d), [Dr]
  Demux/3 -> "J^{-1}"/1(th_c), [Thcr]
  Demux/2 -> [Ycr]
  Demux/1 -> [Xcr]
  Demux3/2 -> [dO1r]
  Demux3/1 -> [O1r]
  Reference Variables/1(Out) -> Demux3/1
  Demux1/4 -> [Y2r]
  Demux1/3 -> [X2r]
  Demux1/2 -> [Y1r]
  Demux1/1 -> [X1r]
  Discrete-Time Integrator 2/1 -> Demux1/1, To Workspace 1/1
  From Workspace 1/1 -> Gain 2/1, Gain 3/1
  [Y2r] -> Reference Robot 2/2
  [X2r] -> Reference Robot 2/1
  [Y1r] -> Reference Robot 1/2
  [X1r] -> Reference Robot 1/1
  Product 1/1 -> Discrete-Time Integrator 2/1, Display 1/1, Demux2/1, Reference Variables/1(In)
  "J^{-1}"/1("J^{-1}") -> Product 1/1
  Demux4/3 -> [dThcr]
  Demux4/4 -> [dDr]
  Demux4/2 -> [dYcr]
  Demux4/1 -> [dXcr]

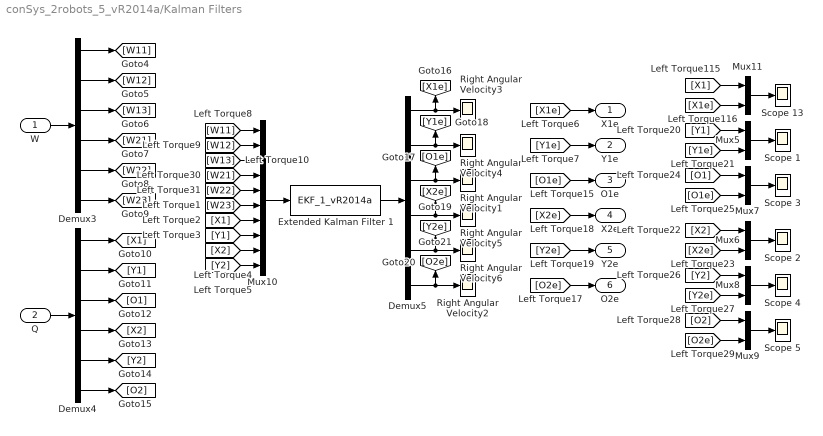
== system conSys_2robots_5_vR2014a/Kalman Filters ==
  W : Inport
  Q : Inport  Port=2
  Demux3 : Demux  Outputs=6
  Demux4 : Demux  Outputs=6
  Demux5 : Demux  Outputs=6
  Extended Kalman Filter 1 : S-Function  FunctionName=EKF_1_vR2014a  Parameters=par  EnableBusSupport=off
  Mux10 : Mux  Inputs=10
  Mux{5..9,11} (6 alike) : Mux  Inputs=2
  Right Angular Velocity{1..6} (6 alike) : Scope
      Right Angular Velocity1 settings: YMin=-3  YMax=6  SaveName=ScopeData5
      Right Angular Velocity2 settings: YMin=-3  YMax=6  SaveName=ScopeData13
      Right Angular Velocity3 settings: YMin=-10000  YMax=10000  SaveName=ScopeData7
      Right Angular Velocity4 settings: YMin=0  YMax=5000  SaveName=ScopeData8
      Right Angular Velocity5 settings: YMin=-10000  YMax=10000  SaveName=ScopeData14
      Right Angular Velocity6 settings: YMin=0  YMax=5000  SaveName=ScopeData15
  Scope {1..5,13} (6 alike) : Scope
      Scope 1 settings: YMin=0  YMax=20000  SaveName=ScopeData29
      Scope 13 settings: YMin=0  YMax=20000  SaveName=ScopeData25
      Scope 2 settings: YMin=-2  YMax=20000  SaveName=ScopeData32
      Scope 3 settings: YMin=-20  YMax=10  SaveName=ScopeData33
      Scope 4 settings: YMin=-2  YMax=20000  SaveName=ScopeData34
      Scope 5 settings: YMin=-20  YMax=10  SaveName=ScopeData35
  X1e : Outport
  Y1e : Outport  Port=2
  O1e : Outport  Port=3
  X2e : Outport  Port=4
  Y2e : Outport  Port=5
  O2e : Outport  Port=6
  wires:
  W/1 -> Demux3/1
  Demux3/1 -> [W11]
  Demux3/2 -> [W12]
  Demux3/3 -> [W13]
  Demux3/4 -> [W21]
  Demux3/5 -> [W22]
  Demux3/6 -> [W23]
  Demux4/1 -> [X1]
  Demux4/2 -> [Y1]
  Demux4/3 -> [O1]
  Demux4/4 -> [X2]
  Demux4/5 -> [Y2]
  Demux4/6 -> [O2]
  Q/1 -> Demux4/1
  [X1e] -> X1e/1
  [Y1e] -> Y1e/1
  [O1e] -> O1e/1
  [X2e] -> X2e/1
  [Y2e] -> Y2e/1
  [O2e] -> O2e/1
  [X1e] -> Mux11/2
  Mux11/1 -> Scope 13/1
  [X1] -> Mux11/1
  [Y1e] -> Mux5/2
  Mux5/1 -> Scope 1/1
  [Y1] -> Mux5/1
  [X2e] -> Mux6/2
  Mux6/1 -> Scope 2/1
  [X2] -> Mux6/1
  [O1e] -> Mux7/2
  Mux7/1 -> Scope 3/1
  [O1] -> Mux7/1
  [Y2e] -> Mux8/2
  Mux8/1 -> Scope 4/1
  [Y2] -> Mux8/1
  [O2e] -> Mux9/2
  Mux9/1 -> Scope 5/1
  [O2] -> Mux9/1
  [W11] -> Mux10/1
  [W12] -> Mux10/2
  [W13] -> Mux10/3
  Mux10/1 -> Extended Kalman Filter 1/1
  Extended Kalman Filter 1/1 -> Demux5/1
  Demux5/2 -> Right Angular Velocity4/1, [Y1e]
  Demux5/3 -> Right Angular Velocity1/1, [O1e]
  Demux5/1 -> Right Angular Velocity3/1, [X1e]
  [W21] -> Mux10/4
  [W22] -> Mux10/5
  Demux5/5 -> [Y2e], Right Angular Velocity6/1
  Demux5/6 -> [O2e], Right Angular Velocity2/1
  Demux5/4 -> [X2e], Right Angular Velocity5/1
  [W23] -> Mux10/6
  [X1] -> Mux10/7
  [Y1] -> Mux10/8
  [Y2] -> Mux10/10
  [X2] -> Mux10/9
